simulink model "model"  (R2025b)
settings: Solver=FixedStepDiscrete  StartTime=0.0  StopTime=inf  RelTol=1e-3
libraries: commdigbbndam3 x2, commchan3 x1, commrandsrc3 x1, commsink2 x1
settings Model: Creator=D.mon  LastModifiedBy=D.mon

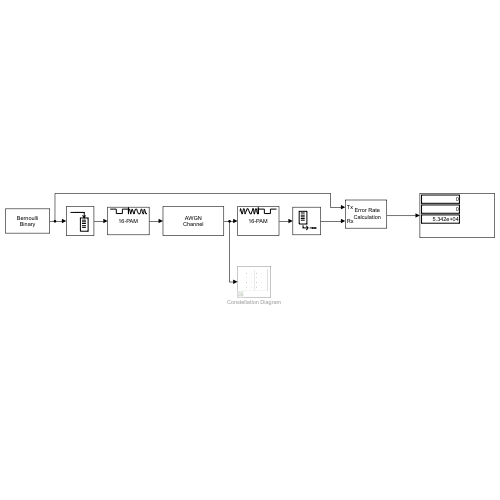
[thumbnail: Simulink's stored preview of the top-level diagram]
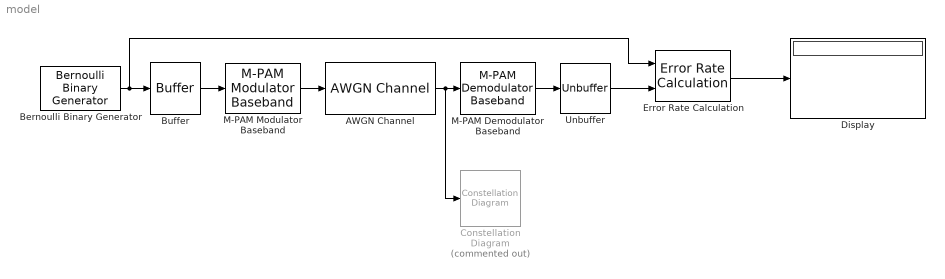
== system model ==
  AWGN Channel : commchan3/AWGN Channel  LegacyMode=off  NoiseMethod="Signal to noise ratio  (Eb/No)"  noiseMode="Signal to noise ratio  (SNR)"  EbNo=inf  EsNo=10  SNR=10  BitsPerSymbol=4  SignalPower=1  SpecifySymbolPeriod=off  SamplesPerSymbol=1  SymbolPeriod=1  VarianceSource=Parameter  Variance=1  RandomStream=mt19937ar with seed  Seed=randi(100000)  SimulateUsing=Code generation
  Bernoulli Binary Generator : commrandsrc3/Bernoulli Binary Generator  ProbabilityOfZero=0.5  SeedSource=Auto  Seed=0  SampleTime=1  SamplesPerFrame=1  OutputDataType=double  SimulateUsing=Interpreted execution
  Buffer : Buffer  N=4  OutputFrames=off
  Constellation Diagram : ConstellationDiagram  Commented=on  WindowPosition=[124.000000,231.000000,600.000000,596.000000,]  ScopeFrameLocation=window  SamplesPerSymbol=4  SymbolsToDisplaySource=Property  SymbolsToDisplay=400  ReferenceConstellation=QPSK  ShowReferenceConstellation=off
  Display : Display
  Error Rate Calculation : commsink2/Error Rate Calculation  N=4  st_delay=0  cp_mode=Entire frame  subframe=[]  PMode=Port  WsName=ErrorVec  RsMode2=off  stop=on  numErr=100  maxBits=1e6
  M-PAM Demodulator Baseband : commdigbbndam3/M-PAM Demodulator Baseband  M=16  OutType=Bit  Dec=Gray  PowType=Average Power  MinDist=2  AvgPow=1  PeakPow=1  outDtype1=Inherit via internal rule  outDtype2=Inherit via internal rule  denormFactorWordLen=16  denormFactorDataTypeStr=Inherit: Same word length as input  denormFactorLastDataTypeStr=Inherit: Same word length as input  prodOutWordLen=16  prodOutRoundingMode=Floor  prodOutOverflowMode=Wrap  prodOutOvFlMode=off  prodOutOvFlModeLastStrValue=off  sumWordLen=16
  M-PAM Modulator Baseband : commdigbbndam3/M-PAM Modulator Baseband  M=16  InType=Bit  Enc=Gray  PowType=Average Power  MinDist=2  AvgPow=1  PeakPow=1  outDtype=double  outWordLen=16  outUDDataType=sfix(16)  outFracLenMode=Best precision  outFracLen=15  outDataTypeStr=double  outLastDataTypeStr=double
  Unbuffer : Unbuffer
  wires:
  Bernoulli Binary Generator/1 -> Error Rate Calculation/1, Buffer/1
  Buffer/1 -> M-PAM Modulator Baseband/1
  M-PAM Modulator Baseband/1 -> AWGN Channel/1
  AWGN Channel/1 -> Constellation Diagram/1, M-PAM Demodulator Baseband/1
  M-PAM Demodulator Baseband/1 -> Unbuffer/1
  Error Rate Calculation/1 -> Display/1
  Unbuffer/1 -> Error Rate Calculation/2
